simulink library "eess_sCap_mhs_std"  (R2016a)
settings: Solver=ode45  StartTime=0.0  StopTime=10.0  RelTol=1e-3
undefined symbols (not defined in the file): sMP
settings Model: Creator=LAUEREL  LastModifiedBy=KNWINDE
settings DataIOCC: LimitDataPoints=on  SaveFormat=Array
settings OptimizationCC: ExpressionDepthLimit=2147483647
settings DebuggingCC: UnderspecifiedInitializationDetection=Classic  MergeDetectMultiDrivingBlocksExec=none  SolverPrmCheckMsg=warning  StateNameClashWarn=warning
settings HardwareCC: ProdBitPerPointer=32  ProdLargestAtomicFloat=None  ProdIntDivRoundTo=Undefined  ProdEndianess=Unspecified  ProdWordSize=32  ProdHWDeviceType=32-bit Generic
settings ModelReferenceCC: PropagateSignalLabelsOutOfModel=off
settings ConfigComp: CovModelRefEnable=Off

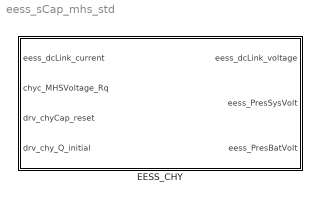
== system eess_sCap_mhs_std ==
  EESS_CHY : Subsystem  mask{MHS_dcdc_Ri_Verpolschutz=sMP.phys.eess.dcdc_Ri_Verpolschutz, MHS_dcdc_U_ZK=sMP.phys.eess.dcdc_U_ZK, MHS_dcdc_U_Cap=sMP.phys.eess.dcdc_U_Cap, MHS_dcdc_I_ZK=sMP.phys.eess.dcdc_I_ZK, MHS_dcdc_Ploss=sMP.phys.eess.dcdc_Ploss, MHS_Ri_Caps=sMP.phys.eess.Ri_Caps, MHS_capacity=sMP.phys.eess.capacity, MHS_nParallel=sMP.phys.eess.nParallel}

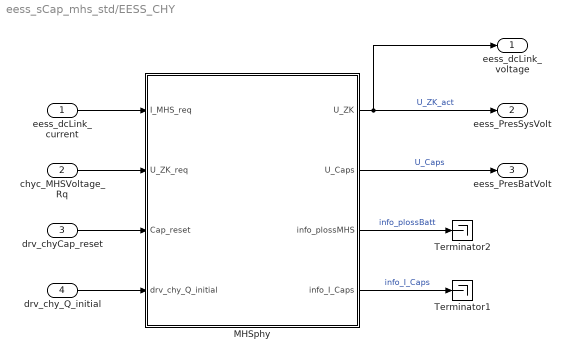
== system eess_sCap_mhs_std/EESS_CHY ==
  eess_dcLink_current : Inport
  chyc_MHSVoltage_Rq : Inport  Port=2
  drv_chyCap_reset : Inport  Port=3
  drv_chy_Q_initial : Inport  Port=4
  MHSphy : Subsystem
  Terminator1 : Terminator
  Terminator2 : Terminator
  eess_dcLink_voltage : Outport  InitialOutput=0
  eess_PresSysVolt : Outport  Port=2  InitialOutput=0
  eess_PresBatVolt : Outport  Port=3  InitialOutput=0
  wires:
  eess_dcLink_current/1 -> MHSphy/1("I_MHS_req ")
  MHSphy/1(U_ZK) -> eess_dcLink_voltage/1, eess_PresSysVolt/1  "U_ZK_act"
  chyc_MHSVoltage_Rq/1 -> MHSphy/2(U_ZK_req)
  MHSphy/4(info_I_Caps) -> Terminator1/1  "info_I_Caps"
  MHSphy/3(info_plossMHS) -> Terminator2/1  "info_plossBatt"
  MHSphy/2(U_Caps) -> eess_PresBatVolt/1  "U_Caps"
  drv_chyCap_reset/1 -> MHSphy/3("Cap_reset ")
  drv_chy_Q_initial/1 -> MHSphy/4(drv_chy_Q_initial)

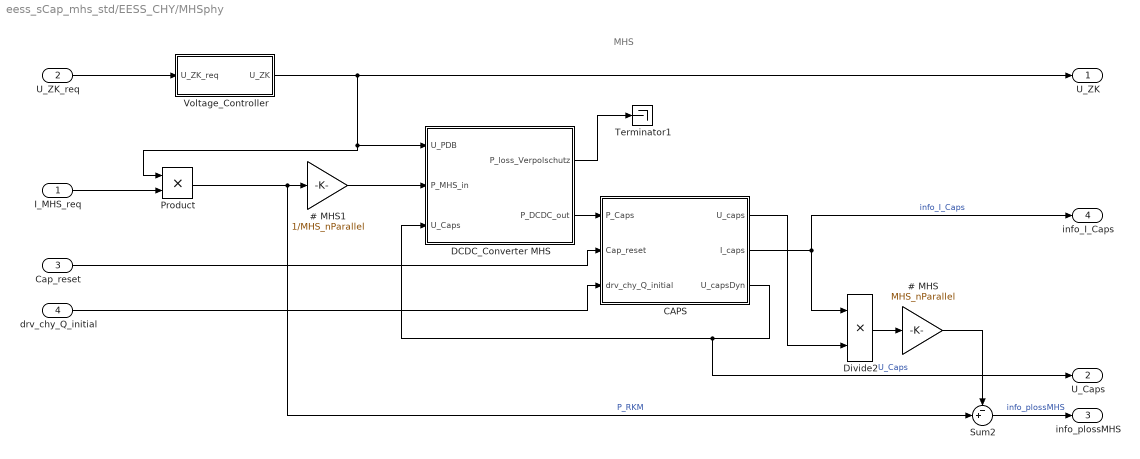
== system eess_sCap_mhs_std/EESS_CHY/MHSphy ==
  note: MHS
  "I_MHS_req " : Inport
  U_ZK_req : Inport  Port=2
  "Cap_reset " : Inport  Port=3
  drv_chy_Q_initial : Inport  Port=4
  # MHS : Gain  Gain=MHS_nParallel
  # MHS1 : Gain  Gain=1/MHS_nParallel
  CAPS : Subsystem
  DCDC_Converter MHS : Subsystem
  Divide2 : Product
  Product : Product  RndMeth=Zero
  Sum2 : Sum  Inputs=-+|
  Terminator1 : Terminator
  Voltage_Controller : Subsystem
  U_ZK : Outport  InitialOutput=0
  U_Caps : Outport  Port=2  InitialOutput=0
  info_plossMHS : Outport  Port=3  InitialOutput=0
  info_I_Caps : Outport  Port=4  InitialOutput=0
  wires:
  Voltage_Controller/1(U_ZK) -> U_ZK/1, DCDC_Converter MHS/1(U_PDB), Product/1
  U_ZK_req/1 -> Voltage_Controller/1(U_ZK_req)
  DCDC_Converter MHS/2(P_DCDC_out) -> CAPS/1(P_Caps)
  CAPS/1(U_caps) -> Divide2/2
  CAPS/2(I_caps) -> Divide2/1, info_I_Caps/1  "info_I_Caps"
  Divide2/1 -> # MHS/1
  # MHS/1 -> Sum2/1
  Sum2/1 -> info_plossMHS/1  "info_plossMHS"
  CAPS/3(U_capsDyn) -> U_Caps/1, DCDC_Converter MHS/3(U_Caps)  "U_Caps"
  Product/1 -> Sum2/2, # MHS1/1  "P_RKM"
  "I_MHS_req "/1 -> Product/2
  # MHS1/1 -> DCDC_Converter MHS/2(P_MHS_in)
  DCDC_Converter MHS/1(P_loss_Verpolschutz) -> Terminator1/1
  "Cap_reset "/1 -> CAPS/2(Cap_reset)
  drv_chy_Q_initial/1 -> CAPS/3(drv_chy_Q_initial)

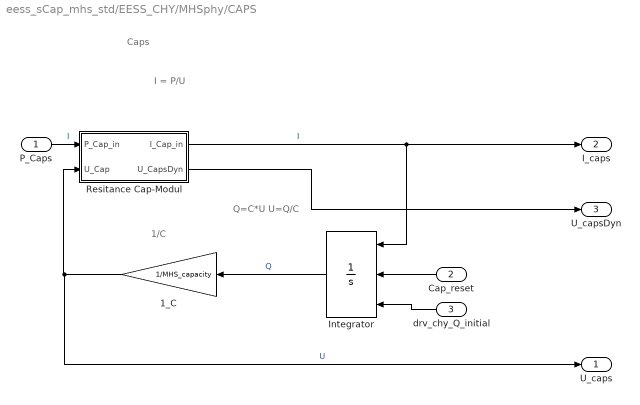
== system eess_sCap_mhs_std/EESS_CHY/MHSphy/CAPS ==
  note: 1/C
  note: Caps
  note: I = P/U
  note: Q=C*U
      | U=Q/C
  P_Caps : Inport
  Cap_reset : Inport  Port=2
  drv_chy_Q_initial : Inport  Port=3
  1_C : Gain  Gain=1/MHS_capacity
  Integrator : Integrator  ExternalReset=rising  InitialConditionSource=external  InitialCondition=(sqrt((0.5*(21.6^2-12^2))+12^2))*750  UpperSaturationLimit=16300  LowerSaturationLimit=-20000
  Resitance Cap-Modul : Subsystem
  U_caps : Outport
  I_caps : Outport  Port=2
  U_capsDyn : Outport  Port=3
  wires:
  drv_chy_Q_initial/1 -> Integrator/3
  Integrator/1 -> 1_C/1  "Q"
  1_C/1 -> U_caps/1, Resitance Cap-Modul/2(U_Cap)  "U"
  Resitance Cap-Modul/1(I_Cap_in) -> Integrator/1, I_caps/1  "I"
  P_Caps/1 -> Resitance Cap-Modul/1(P_Cap_in)  "I"
  Resitance Cap-Modul/2(U_CapsDyn) -> U_capsDyn/1
  Cap_reset/1 -> Integrator/2

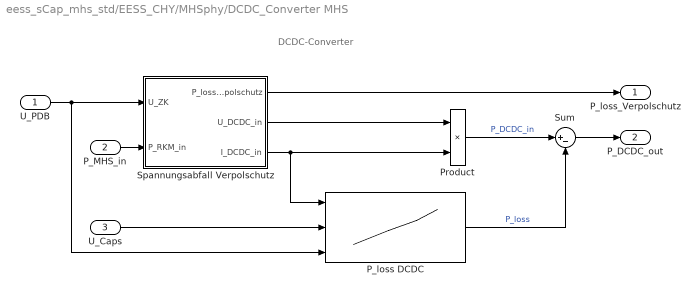
== system eess_sCap_mhs_std/EESS_CHY/MHSphy/DCDC_Converter MHS ==
  note: DCDC-Converter
  U_PDB : Inport
  P_MHS_in : Inport  Port=2
  U_Caps : Inport  Port=3
  P_loss DCDC : Lookup_n-D  NumberOfTableDimensions=3  BreakpointsForDimension1=MHS_dcdc_I_ZK  BreakpointsForDimension2=MHS_dcdc_U_Cap  BreakpointsForDimension3=MHS_dcdc_U_ZK  Table=MHS_dcdc_Ploss  RndMeth=Simplest  InputSameDT=on
  Product : Product  RndMeth=Zero
  Spannungsabfall Verpolschutz : Subsystem
  Sum : Sum  Inputs=|+-
  P_loss_Verpolschutz : Outport
  P_DCDC_out : Outport  Port=2
  wires:
  Spannungsabfall Verpolschutz/1(P_loss_Verpolschutz) -> P_loss_Verpolschutz/1
  Sum/1 -> P_DCDC_out/1
  P_loss DCDC/1 -> Sum/2  "P_loss"
  Spannungsabfall Verpolschutz/2(U_DCDC_in) -> Product/1
  Spannungsabfall Verpolschutz/3(I_DCDC_in) -> Product/2, P_loss DCDC/1
  P_MHS_in/1 -> Spannungsabfall Verpolschutz/2(P_RKM_in)
  U_PDB/1 -> Spannungsabfall Verpolschutz/1(U_ZK), P_loss DCDC/3
  Product/1 -> Sum/1  "P_DCDC_in"
  U_Caps/1 -> P_loss DCDC/2

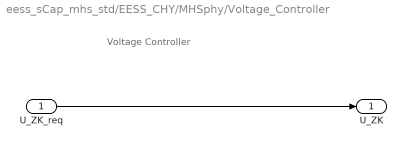
== system eess_sCap_mhs_std/EESS_CHY/MHSphy/Voltage_Controller ==
  note: Voltage Controller
  U_ZK_req : Inport
  U_ZK : Outport
  wires:
  U_ZK_req/1 -> U_ZK/1

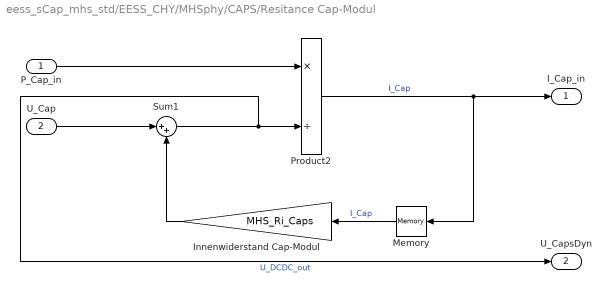
== system eess_sCap_mhs_std/EESS_CHY/MHSphy/CAPS/Resitance Cap-Modul ==
  P_Cap_in : Inport
  U_Cap : Inport  Port=2
  Innenwiderstand Cap-Modul : Gain  Gain=MHS_Ri_Caps
  Memory : Memory
  Product2 : Product  Inputs=*/  RndMeth=Zero
  Sum1 : Sum  Inputs=|++
  I_Cap_in : Outport
  U_CapsDyn : Outport  Port=2
  wires:
  P_Cap_in/1 -> Product2/1
  Innenwiderstand Cap-Modul/1 -> Sum1/2
  Memory/1 -> Innenwiderstand Cap-Modul/1  "I_Cap"
  U_Cap/1 -> Sum1/1
  Product2/1 -> Memory/1, I_Cap_in/1  "I_Cap"
  Sum1/1 -> U_CapsDyn/1, Product2/2  "U_DCDC_out"

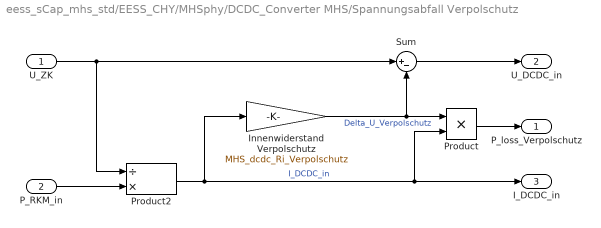
== system eess_sCap_mhs_std/EESS_CHY/MHSphy/DCDC_Converter MHS/Spannungsabfall Verpolschutz ==
  U_ZK : Inport
  P_RKM_in : Inport  Port=2
  Innenwiderstand Verpolschutz : Gain  Gain=MHS_dcdc_Ri_Verpolschutz
  Product : Product  RndMeth=Zero
  Product2 : Product  Inputs=/*  RndMeth=Zero
  Sum : Sum  Inputs=|+-
  P_loss_Verpolschutz : Outport
  U_DCDC_in : Outport  Port=2
  I_DCDC_in : Outport  Port=3
  wires:
  Product/1 -> P_loss_Verpolschutz/1
  Product2/1 -> Product/2, I_DCDC_in/1, Innenwiderstand Verpolschutz/1  "I_DCDC_in"
  P_RKM_in/1 -> Product2/2
  Innenwiderstand Verpolschutz/1 -> Product/1, Sum/2  "Delta_U_Verpolschutz"
  U_ZK/1 -> Sum/1, Product2/1
  Sum/1 -> U_DCDC_in/1
